simulink model "KITTdynamics"  (R2021a)
settings: Solver=VariableStepAuto  StartTime=0.0  StopTime=50  RelTol=1e-3
values from neighbouring files (symbols this model uses):
  b = 0.0015    [KITTVelocity.m]    (also in KITTparameters.m)
  c = 0.02    [KITTVelocity.m]    (also in KITTparameters.m)
  m = 13    [KITTVelocity.m]    (also in KITTparameters.m; structure_car.m = 5.6)
settings Model: Creator=meath  LastModifiedBy=meath

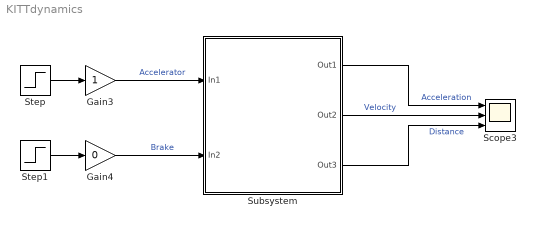
== system KITTdynamics ==
  Gain3 : Gain
  Gain4 : Gain  Gain=0
  Scope3 : Scope  NumInputPorts=3
  Step : Step  After=80  SampleTime=0
  Step1 : Step  After=120  SampleTime=0
  Subsystem : Subsystem
  wires:
  Step/1 -> Gain3/1
  Step1/1 -> Gain4/1
  Gain3/1 -> Subsystem/1(In1)  "Accelerator"
  Gain4/1 -> Subsystem/2(In2)  "Brake"
  Subsystem/1(Out1) -> Scope3/1  "Acceleration"
  Subsystem/2(Out2) -> Scope3/2  "Velocity"
  Subsystem/3(Out3) -> Scope3/3  "Distance"

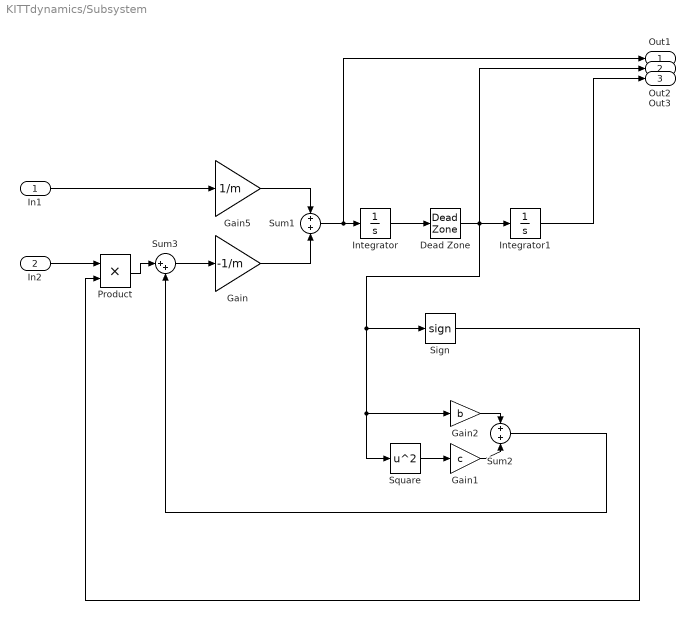
== system KITTdynamics/Subsystem ==
  In1 : Inport
  In2 : Inport  Port=2
  Dead Zone : DeadZone  LowerValue=-0.05  UpperValue=0.05  ZeroCross=off  SaturateOnIntegerOverflow=on
  Gain : Gain  Gain=-1/m
  Gain1 : Gain  Gain=c
  Gain2 : Gain  Gain=b
  Gain5 : Gain  Gain=1/m
  Integrator : Integrator
  Integrator1 : Integrator
  Product : Product
  Sign : Signum  ZeroCross=off
  Square : Math  Operator=square  SaturateOnIntegerOverflow=on
  Sum1 : Sum  Inputs=+|+
  Sum2 : Sum  Inputs=+|+
  Sum3 : Sum  Inputs=|++
  Out1 : Outport
  Out2 : Outport  Port=2
  Out3 : Outport  Port=3
  wires:
  Sum1/1 -> Out1/1, Integrator/1
  Integrator1/1 -> Out3/1
  Gain1/1 -> Sum2/2
  Dead Zone/1 -> Out2/1, Sign/1, Gain2/1, Square/1, Integrator1/1
  Sum3/1 -> Gain/1
  Gain2/1 -> Sum2/1
  Sum2/1 -> Sum3/2
  Sign/1 -> Product/2
  Product/1 -> Sum3/1
  Gain/1 -> Sum1/2
  Square/1 -> Gain1/1
  Gain5/1 -> Sum1/1
  Integrator/1 -> Dead Zone/1
  In1/1 -> Gain5/1
  In2/1 -> Product/1
